simulink library "Susp_TwistBeam"  (R2025b)
settings: Solver=VariableStepAuto  StartTime=0.0  StopTime=10.0  RelTol=1e-3
undefined symbols (not defined in the file): Axle1D, AxleIn, Init, RaceFix, RaceSpin, TwistBeam, Visual, X, Y, Z
libraries: sm_lib x30, Suspension_Utilities x14, Linkage_Shock x2, fl_lib x2, nesl_utility x2, Linkage_Spring x2, Susp_TwistBeam_Components x2
(part 1 of 2)
Description:
  | Component of Simscape Vehicle Templates Library
  | 
  | Copyright 2018-2024 The MathWorks, Inc.
settings Model: Creator=mwalker  LastModifiedBy=smiller
settings SolverCC: AlgebraicLoopSolver=TrustRegion
settings DataIOCC: ReturnWorkspaceOutputs=off
settings DebuggingCC: UnconnectedInputMsg=warning  UnconnectedOutputMsg=warning  UnconnectedLineMsg=warning  ArithmeticOperatorsInVariantConditions=warning
settings ModelReferenceCC: EnableRefExpFcnMdlSchedulingChecks=on
settings SFSimCC: CustomCodeUndefinedFunction=UseInterfaceOnly
settings RTWCC: GPUComputeCapability=3.5

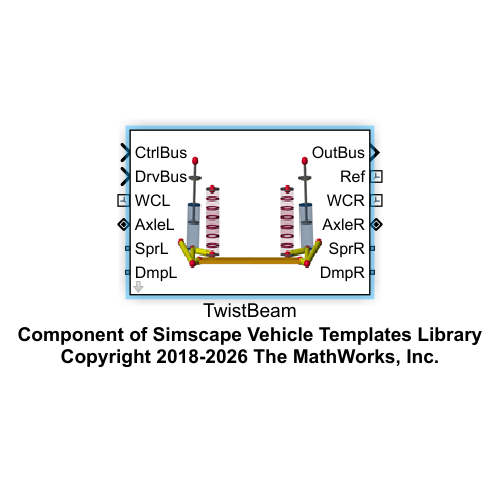
[thumbnail: Simulink's stored preview of the top-level diagram]
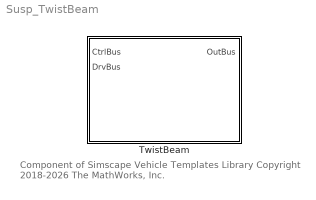
== system Susp_TwistBeam ==
  note: Component of Simscape Vehicle Templates Library
      | Copyright 2018-2026 The MathWorks, Inc.
  TwistBeam : Subsystem  VariantControl=LiveAxle  mask(Twist Beam Suspension){Init=Init.Axle2, hp_arm=TwistBeam.TrailingArm.sBody.Value, hp_dmp_top=TwistBeam.Damper.sTop.Value, hp_dmp_bot=TwistBeam.Damper.sBottom.Value, hp_spr_top=TwistBeam.Spring.sTop.Value, hp_spr_bot=TwistBeam.Spring.sBottom.Value, hp_beam=TwistBeam.Beam.sOutboard.Value, hp_whl_ctr=TwistBeam.TrailingArm.sWheelCentre.Value, Arm_to_Subframe=TwistBeam.Arm_to_Subframe, Damper_to_Subframe=TwistBeam.Damper_to_Subframe, Damper_to_Arm=TwistBeam.Damper_to_Arm, arm_mass=TwistBeam.TrailingArm.m.Value, axle_mass=TwistBeam.TrailingArm.mAxle.Value, axle_len=TwistBeam.TrailingArm.xAxle.Value, axle_whlc_to_bearing=TwistBeam.TrailingArm.xWCtoBearing.Value, beam_rho=TwistBeam.Beam.density.Value, beam_E=TwistBeam.Beam.E.Value, beam_nu=TwistBeam.Beam.nu.Value, beam_zeta=TwistBeam.Beam.zDamping.Value, xc_x=TwistBeam.Beam.xcX.Value, xc_z=TwistBeam.Beam.xcZ.Value, beam_numElements=TwistBeam.Beam.numElements.Value, opc_beam=Visual.part.opc, clr_beam=Visual.clr.orangedark, radius_axle=Visual.Axle.rad, clr_axle=Visual.Axle.clr, opc_axle=Visual.part.opc, clr_upr=Visual.UpperArm.clr, opc_upr=Visual.part.opc, piston_mass=TwistBeam.Shock.mPiston.Value, cyl_mass=TwistBeam.Shock.mCylinder.Value, damper_xmax=TwistBeam.Endstop.xMax.Value, damper_xmin=TwistBeam.Endstop.xMin.Value, spring_mass=TwistBeam.Spring.m.Value}
      mask prompts: Init "Initial Wheel Speed (rad/s)"; hp_arm "HP Arm to Body [xyz] (m)"; hp_dmp_top "HP Damper Top [xyz] (m)"; hp_dmp_bot "HP Damper Bottom [xyz] (m)"; hp_spr_top "HP Spring Top [xyz] (m)"; hp_spr_bot "HP Spring Bottom [xyz] (m)"; hp_beam "HP Beam Outboard [xyz] (m)"; hp_whl_ctr "HP Wheel Center [xyz] (m)"; Arm_to_Subframe "Arm to Subframe Connection (structure)"; Damper_to_Subframe "Damper to Subframe Connection"; Damper_to_Arm "Damper to Arm Connection"; arm_mass "Arm Mass (kg)"; axle_mass "Axle Mass (kg)"; axle_len "Axle Length (m)"; axle_whlc_to_bearing "Distance Wheel Ctr to Bearing (m)"; beam_rho "Beam Density (kg/m^3)"; beam_E "Young's Modulus (GPa)"; beam_nu "Poisson's Ratio"; beam_zeta "Damping Constant (sec)"; xc_x "Extrusion Points X (m)"; xc_z "Extrusion Points Z (m)"; beam_numElements "Number of Beam Elements"; opc_beam "Beam Opacity (0-1)"; clr_beam "Beam Color [RGB]"; radius_axle "Axle Radius (m)"; clr_axle "Axle Color [RGB]"; opc_axle "Axle Opacity (0-1)"; clr_upr "Bearing Color [RGB]"; opc_upr "Bearing Opacity (0-1)"; piston_mass "Piston Mass (kg)"; cyl_mass "Cylinder Mass (kg)"; damper_xmax "Upper Limit Bumpstop (m)"; damper_xmin "Lower Limit Bumpstop (m)"; spring_mass "Spring Mass (kg)"
      mask help: Models a twist beam suspension with independent connections for dampers and springs.
      mask TypeOptions axle_whlc_to_bearing:
      | Transform
      | sWheelCtrL/TranslationStandardOffset | Transform
      | sWheelCtrR/TranslationStandardOffset | Trailing
      | Arm L/axle_whlc_to_bearing | Trailing
      | Arm R/axle_whlc_to_bearing
      mask TypeOptions beam_rho: Beam/beam_rho
      mask TypeOptions beam_E: Beam/beam_E
      mask TypeOptions beam_nu: Beam/beam_nu
      mask TypeOptions beam_zeta: Beam/beam_zeta
      mask TypeOptions xc_x: Beam/xc_x
      mask TypeOptions xc_z: Beam/xc_z
      mask TypeOptions beam_numElements: Beam/beam_numElements
      mask TypeOptions opc_beam: Beam/opc_beam
      mask TypeOptions clr_beam: Beam/clr_beam
      mask DialogControl Container4 Prompt: Hardpoints
      mask DialogControl Container5 Prompt: Parts
      mask DialogControl Container7 Prompt: Visualization
      mask DialogControl Container6 Prompt: Shock
      mask Display: image('sm_car_vehicle_susp_twistbeam_IMAGE.png');

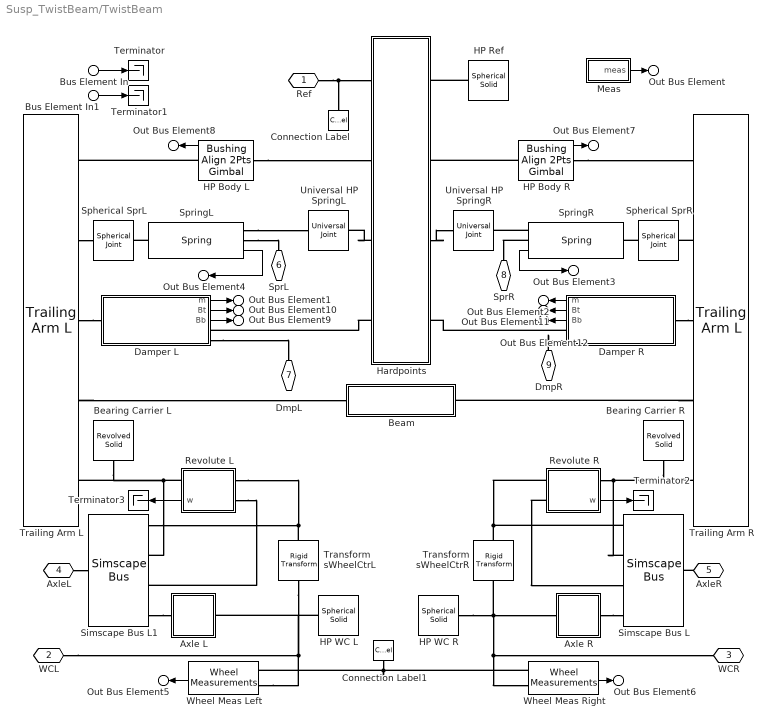
== system Susp_TwistBeam/TwistBeam ==
  Bus Element In1 : Inport  PortName=CtrlBus
  Bus Element In : Inport  Port=2  PortName=DrvBus
  Axle L : Subsystem
  Axle R : Subsystem
  Beam : Subsystem  mask(Leaf spring){popup_leftRight=Left, hp_beam=hp_beam, beam_rho=beam_rho, xc_x=xc_x, xc_z=xc_z, beam_E=beam_E, beam_nu=beam_nu, beam_zeta=beam_zeta, beam_numElements=beam_numElements, clr_beam=clr_beam, opc_beam=opc_beam}
      mask prompts: popup_leftRight "Left/Right"; hp_beam "HP Beam [xyz] (m)"; beam_rho "Beam Density (kg/m^3)"; xc_x "Extrusion Points X (m)"; xc_z "Extrusion Points Z (m)"; beam_E "Young's Modulus (GPa)"; beam_nu "Poisson's Ratio"; beam_zeta "Damping Constant (sec)"; beam_numElements "Number of Beam Elements"; clr_beam "Beam Color [RGB]"; opc_beam "Beam Opacity (0-1)"
      mask help: Models leaf spring using flexible body.
      mask init:
      | if(popup_leftRight == 1)
      |     rhs_susp = [1 1 1];
      | elseif(popup_leftRight == 2)
      |     rhs_susp = [1 -1 1];
      | end
      | 
      | beam_len = hp_beam(2)*2;
      mask TypeOptions popup_leftRight: Left | Right
      mask DialogControl cont_vis Prompt: Visualization
      mask Display: image('sm_car_vehicle_susp_leaf_spring_IMAGE.png')
  Bearing Carrier L : sm_lib/Body Elements/Revolved Solid  RevolutionCrossSection=[1.2 0.5;1.1 0.5;1.1 -0.5;1.2 -0.5].*[radius_axle 0.05]  RevolutionCrossSectionUnits=m  RevolutionExtent=Full  RevolutionAngle=180  RevolutionAngleUnits=deg  ExportConvexHullGeometry=off  InertiaType=CalculateFromGeometry  BasedOnType=Density  Density=1000  DensityUnits=kg/m^3  Mass=1  MassUnits=kg  CenterOfMass=[0 0 0]  CenterOfMassUnits=m  MomentsOfInertia=[1 1 1]  MomentsOfInertiaUnits=kg*m^2  ProductsOfInertia=[0 0 0]  ProductsOfInertiaUnits=kg*m^2  GraphicType=FromGeometry  MarkerShape=Sphere  MarkerSize=10  GraphicVisPropType=SimpleVisualProperties  GraphicDiffuseColor=clr_upr  GraphicOpacity=0.5  GraphicSpecularColor=[0.5 0.5 0.5 1.0]  GraphicAmbientColor=[0.15 0.15 0.15 1.0]  GraphicEmissiveColor=[0.0 0.0 0.0 1.0]  GraphicShininess=75  DoExposeReferenceFrame=on  SerializedFrames=<Frames/>
  Bearing Carrier R : sm_lib/Body Elements/Revolved Solid  RevolutionCrossSection=[1.2 0.5;1.1 0.5;1.1 -0.5;1.2 -0.5].*[radius_axle 0.05]  RevolutionCrossSectionUnits=m  RevolutionExtent=Full  RevolutionAngle=180  RevolutionAngleUnits=deg  ExportConvexHullGeometry=off  InertiaType=CalculateFromGeometry  BasedOnType=Density  Density=1000  DensityUnits=kg/m^3  Mass=1  MassUnits=kg  CenterOfMass=[0 0 0]  CenterOfMassUnits=m  MomentsOfInertia=[1 1 1]  MomentsOfInertiaUnits=kg*m^2  ProductsOfInertia=[0 0 0]  ProductsOfInertiaUnits=kg*m^2  GraphicType=FromGeometry  MarkerShape=Sphere  MarkerSize=10  GraphicVisPropType=SimpleVisualProperties  GraphicDiffuseColor=clr_upr  GraphicOpacity=0.5  GraphicSpecularColor=[0.5 0.5 0.5 1.0]  GraphicAmbientColor=[0.15 0.15 0.15 1.0]  GraphicEmissiveColor=[0.0 0.0 0.0 1.0]  GraphicShininess=75  DoExposeReferenceFrame=on  SerializedFrames=<Frames/>
  Connection Label : ConnectionLabel  Label=Ref
  Connection Label1 : ConnectionLabel  Label=Ref
  Damper L : Subsystem
      mask Display: image('sm_car_vehicle_linkage_shock_IMAGE.png');
  Damper R : Subsystem
      mask Display: image('sm_car_vehicle_linkage_shock_IMAGE.png');
  HP Body L : Suspension_Utilities/Bushing Align 2Pts Gimbal  VariantControl=Variant1  LabelModeActiveChoice=Bushing_Tr3Ro3  popup_leftRight=Left  hp_joint=hp_arm  Connection=Arm_to_Subframe  VariantLabel=Arm_to_Subframe.class.Value  checkbox_setTargets=off
      settings: AttributesFormatString=%<ActiveVariant>
  HP Body R : Suspension_Utilities/Bushing Align 2Pts Gimbal  VariantControl=Variant1  LabelModeActiveChoice=Bushing_Tr3Ro3  popup_leftRight=Right  hp_joint=hp_arm  Connection=Arm_to_Subframe  VariantLabel=Arm_to_Subframe.class.Value  checkbox_setTargets=off
      settings: AttributesFormatString=%<ActiveVariant>
  HP Ref : sm_lib/Body Elements/Spherical Solid  SphereRadius=Visual.hp.rad  SphereRadiusUnits=m  ExportEntireGeometry=off  InertiaType=CalculateFromGeometry  BasedOnType=Density  Density=1000  DensityUnits=kg/m^3  Mass=1  MassUnits=kg  CenterOfMass=[0 0 0]  CenterOfMassUnits=m  MomentsOfInertia=[1 1 1]  MomentsOfInertiaUnits=kg*m^2  ProductsOfInertia=[0 0 0]  ProductsOfInertiaUnits=kg*m^2  GraphicType=FromGeometry  MarkerShape=Sphere  MarkerSize=10  GraphicVisPropType=SimpleVisualProperties  GraphicDiffuseColor=Visual.hp.clr  GraphicOpacity=Visual.hp.opc  GraphicSpecularColor=[0.5 0.5 0.5 1.0]  GraphicAmbientColor=[0.15 0.15 0.15 1.0]  GraphicEmissiveColor=[0.0 0.0 0.0 1.0]  GraphicShininess=75  DoExposeReferenceFrame=on  SerializedFrames=<Frames/>
  HP WC L : sm_lib/Body Elements/Spherical Solid  SphereRadius=Visual.hp.rad  SphereRadiusUnits=m  ExportEntireGeometry=off  InertiaType=CalculateFromGeometry  BasedOnType=Density  Density=1000  DensityUnits=kg/m^3  Mass=1  MassUnits=kg  CenterOfMass=[0 0 0]  CenterOfMassUnits=m  MomentsOfInertia=[1 1 1]  MomentsOfInertiaUnits=kg*m^2  ProductsOfInertia=[0 0 0]  ProductsOfInertiaUnits=kg*m^2  GraphicType=FromGeometry  MarkerShape=Sphere  MarkerSize=10  GraphicVisPropType=SimpleVisualProperties  GraphicDiffuseColor=Visual.hp.clr  GraphicOpacity=Visual.hp.opc  GraphicSpecularColor=[0.5 0.5 0.5 1.0]  GraphicAmbientColor=[0.15 0.15 0.15 1.0]  GraphicEmissiveColor=[0.0 0.0 0.0 1.0]  GraphicShininess=75  DoExposeReferenceFrame=on  SerializedFrames=<Frames/>
  HP WC R : sm_lib/Body Elements/Spherical Solid  SphereRadius=Visual.hp.rad  SphereRadiusUnits=m  ExportEntireGeometry=off  InertiaType=CalculateFromGeometry  BasedOnType=Density  Density=1000  DensityUnits=kg/m^3  Mass=1  MassUnits=kg  CenterOfMass=[0 0 0]  CenterOfMassUnits=m  MomentsOfInertia=[1 1 1]  MomentsOfInertiaUnits=kg*m^2  ProductsOfInertia=[0 0 0]  ProductsOfInertiaUnits=kg*m^2  GraphicType=FromGeometry  MarkerShape=Sphere  MarkerSize=10  GraphicVisPropType=SimpleVisualProperties  GraphicDiffuseColor=Visual.hp.clr  GraphicOpacity=Visual.hp.opc  GraphicSpecularColor=[0.5 0.5 0.5 1.0]  GraphicAmbientColor=[0.15 0.15 0.15 1.0]  GraphicEmissiveColor=[0.0 0.0 0.0 1.0]  GraphicShininess=75  DoExposeReferenceFrame=on  SerializedFrames=<Frames/>
  Hardpoints : Subsystem
  Meas : Subsystem
  Revolute L : Subsystem  mask{whl_spd_init_jnt=Init.nWheel.Value(1)}
      mask prompts: whl_spd_init_jnt "Initial Wheel Speed (rad/s)"
      mask Display: image('sm_car_variant_revolute.png')
  Revolute R : Subsystem  mask{whl_spd_init_jnt=Init.nWheel.Value(2)}
      mask prompts: whl_spd_init_jnt "Initial Wheel Speed (rad/s)"
      mask Display: image('sm_car_variant_revolute.png')
  Simscape Bus L : SimscapeBus  HierarchyStrings=RaceSpin;RaceFix;Axle1D;AxleIn
  Simscape Bus L1 : SimscapeBus  HierarchyStrings=RaceSpin;RaceFix;Axle1D;AxleIn
  Spherical SprL : sm_lib/Joints/Spherical Joint  JointMode=Normal  CompositeWrenchDir=FollowerOnBase  CompositeWrenchFrame=BaseFrame  SenseConstraintForce=off  SenseConstraintTorque=off  SenseTotalForce=off  SenseTotalTorque=off  PositionTargetSpecify=off  PositionTargetPriority=High  PositionTargetRotationMethod=None  PositionTargetFollAlignAxisA=+X  PositionTargetBaseAlignAxisA=+Y  PositionTargetFollAlignAxisB=+Y  PositionTargetBaseAlignAxisB=+Z  PositionTargetRotationStandardAxis=+Z  PositionTargetRotationAngle=0.0  PositionTargetRotationAngleUnits=deg  PositionTargetRotationArbitraryAxis=[0 0 1]  PositionTargetRotationSequenceAxes=FollowerAxes  PositionTargetRotationSequence=XYX  PositionTargetRotationSequenceAngles=[0 0 0]  PositionTargetRotationSequenceAnglesUnits=deg  PositionTargetRotationMatrix=[1 0 0; 0 1 0; 0 0 1]  PositionTargetQuaternion=[1 0 0 0]  VelocityTargetSpecify=off  VelocityTargetPriority=High  VelocityTargetValue=[0 0 0]  VelocityTargetValueUnits=deg/s  VelocityTargetInFollowerFrame=on  EqPosRotationMethod=None  EqPosFollAlignAxisA=+X  EqPosBaseAlignAxisA=+Y  EqPosFollAlignAxisB=+Y  EqPosBaseAlignAxisB=+Z  EqPosRotationStandardAxis=+Z  EqPosRotationAngle=0.0  EqPosRotationAngleUnits=deg  EqPosRotationArbitraryAxis=[0 0 1]  EqPosRotationSequenceAxes=FollowerAxes  EqPosRotationSequence=XYX  EqPosRotationSequenceAngles=[0 0 0]  EqPosRotationSequenceAnglesUnits=deg  EqPosRotationMatrix=[1 0 0; 0 1 0; 0 0 1]  EqPosQuaternion=[1 0 0 0]  SpringStiffness=0  SpringStiffnessUnits=N*m/deg  DampingCoefficient=0  DampingCoefficientUnits=N*m/(deg/s)  LowerLimitSpecify=off  LowerLimitBound=15  LowerLimitBoundUnits=deg  LowerLimitStiffness=1e4  LowerLimitStiffnessUnits=N*m/deg  LowerLimitDamping=10  LowerLimitDampingUnits=N*m/(deg/s)  LowerLimitTransitionRegionWidth=0.1  LowerLimitTransitionRegionWidthUnits=deg  UpperLimitSpecify=off  UpperLimitBound=45  UpperLimitBoundUnits=deg  UpperLimitStiffness=1e4  UpperLimitStiffnessUnits=N*m/deg  UpperLimitDamping=10  UpperLimitDampingUnits=N*m/(deg/s)  UpperLimitTransitionRegionWidth=0.1  UpperLimitTransitionRegionWidthUnits=deg  TorqueActuationMode=NoTorque  ActuateTorqueX=off  ActuateTorqueY=off  ActuateTorqueZ=off  ActuateTorque=off  ActuationFrame=BaseFrame  SensePosition=off  SenseVelocityX=off  SenseVelocityY=off  SenseVelocityZ=off  SenseVelocity=off  SenseAccelerationX=off  SenseAccelerationY=off  SenseAccelerationZ=off  SenseAcceleration=off  SenseLowerLimitTorqueMag=off  SenseUpperLimitTorqueMag=off  SensingFrame=BaseFrame
  Spherical SprR : sm_lib/Joints/Spherical Joint  JointMode=Normal  CompositeWrenchDir=FollowerOnBase  CompositeWrenchFrame=BaseFrame  SenseConstraintForce=off  SenseConstraintTorque=off  SenseTotalForce=off  SenseTotalTorque=off  PositionTargetSpecify=off  PositionTargetPriority=High  PositionTargetRotationMethod=None  PositionTargetFollAlignAxisA=+X  PositionTargetBaseAlignAxisA=+Y  PositionTargetFollAlignAxisB=+Y  PositionTargetBaseAlignAxisB=+Z  PositionTargetRotationStandardAxis=+Z  PositionTargetRotationAngle=0.0  PositionTargetRotationAngleUnits=deg  PositionTargetRotationArbitraryAxis=[0 0 1]  PositionTargetRotationSequenceAxes=FollowerAxes  PositionTargetRotationSequence=XYX  PositionTargetRotationSequenceAngles=[0 0 0]  PositionTargetRotationSequenceAnglesUnits=deg  PositionTargetRotationMatrix=[1 0 0; 0 1 0; 0 0 1]  PositionTargetQuaternion=[1 0 0 0]  VelocityTargetSpecify=off  VelocityTargetPriority=High  VelocityTargetValue=[0 0 0]  VelocityTargetValueUnits=deg/s  VelocityTargetInFollowerFrame=on  EqPosRotationMethod=None  EqPosFollAlignAxisA=+X  EqPosBaseAlignAxisA=+Y  EqPosFollAlignAxisB=+Y  EqPosBaseAlignAxisB=+Z  EqPosRotationStandardAxis=+Z  EqPosRotationAngle=0.0  EqPosRotationAngleUnits=deg  EqPosRotationArbitraryAxis=[0 0 1]  EqPosRotationSequenceAxes=FollowerAxes  EqPosRotationSequence=XYX  EqPosRotationSequenceAngles=[0 0 0]  EqPosRotationSequenceAnglesUnits=deg  EqPosRotationMatrix=[1 0 0; 0 1 0; 0 0 1]  EqPosQuaternion=[1 0 0 0]  SpringStiffness=0  SpringStiffnessUnits=N*m/deg  DampingCoefficient=0  DampingCoefficientUnits=N*m/(deg/s)  LowerLimitSpecify=off  LowerLimitBound=15  LowerLimitBoundUnits=deg  LowerLimitStiffness=1e4  LowerLimitStiffnessUnits=N*m/deg  LowerLimitDamping=10  LowerLimitDampingUnits=N*m/(deg/s)  LowerLimitTransitionRegionWidth=0.1  LowerLimitTransitionRegionWidthUnits=deg  UpperLimitSpecify=off  UpperLimitBound=45  UpperLimitBoundUnits=deg  UpperLimitStiffness=1e4  UpperLimitStiffnessUnits=N*m/deg  UpperLimitDamping=10  UpperLimitDampingUnits=N*m/(deg/s)  UpperLimitTransitionRegionWidth=0.1  UpperLimitTransitionRegionWidthUnits=deg  TorqueActuationMode=NoTorque  ActuateTorqueX=off  ActuateTorqueY=off  ActuateTorqueZ=off  ActuateTorque=off  ActuationFrame=BaseFrame  SensePosition=off  SenseVelocityX=off  SenseVelocityY=off  SenseVelocityZ=off  SenseVelocity=off  SenseAccelerationX=off  SenseAccelerationY=off  SenseAccelerationZ=off  SenseAcceleration=off  SenseLowerLimitTorqueMag=off  SenseUpperLimitTorqueMag=off  SensingFrame=BaseFrame
  SpringL : Linkage_Spring/Spring  spring_mass=spring_mass  hp_spr_top=hp_spr_top  hp_spr_bot=hp_spr_bot  clr_conn_shock=Visual.hp.clr  opc_conn_shock=Visual.hp.opc  size_conn_shock=Visual.hp.rad  clr_spring_cyl=Visual.Spring.cyl.clr  opc_shock_cyl=Visual.Spring.cyl.opc  radius_shock_cyl=0.05  clr_spring_cap=Visual.Spring.cap.clr  opc_spring_cap=Visual.part.opc  clr_spring_coil=Visual.Spring.coil.clr  opc_spring_coil=Visual.Spring.coil.opc  cyl_cap_len_shock=Visual.Shock.cap.len
  SpringR : Linkage_Spring/Spring  spring_mass=spring_mass  hp_spr_top=hp_spr_top  hp_spr_bot=hp_spr_bot  clr_conn_shock=Visual.hp.clr  opc_conn_shock=Visual.hp.opc  size_conn_shock=Visual.hp.rad  clr_spring_cyl=Visual.Spring.cyl.clr  opc_shock_cyl=Visual.Spring.cyl.opc  radius_shock_cyl=0.05  clr_spring_cap=Visual.Spring.cap.clr  opc_spring_cap=Visual.part.opc  clr_spring_coil=Visual.Spring.coil.clr  opc_spring_coil=Visual.Spring.coil.opc  cyl_cap_len_shock=Visual.Shock.cap.len
  Terminator{,1..3} (4 alike) : Terminator
  Trailing Arm L : Susp_TwistBeam_Components/Trailing Arm L  VariantControl=Steer  popup_leftRight=Left  hp_body=hp_arm  hp_spr_bot=hp_spr_bot  hp_dam_bot=hp_dmp_bot  hp_wctr=hp_whl_ctr  hp_beam=hp_beam  axle_whlc_to_bearing=axle_whlc_to_bearing  rod_mass=arm_mass  clr_conn_rod=Visual.hp.clr  opc_conn_rod=Visual.hp.opc  size_conn_rod=Visual.hp.rad  clr_rod=Visual.UpperArm.clr  opc_rod=Visual.part.opc  radius_rod=Visual.UpperArm.rad
  Trailing Arm R : Susp_TwistBeam_Components/Trailing Arm L  VariantControl=Steer  popup_leftRight=Right  hp_body=hp_arm  hp_spr_bot=hp_spr_bot  hp_dam_bot=hp_dmp_bot  hp_wctr=hp_whl_ctr  hp_beam=hp_beam  axle_whlc_to_bearing=axle_whlc_to_bearing  rod_mass=arm_mass  clr_conn_rod=Visual.hp.clr  opc_conn_rod=Visual.hp.opc  size_conn_rod=Visual.hp.rad  clr_rod=Visual.UpperArm.clr  opc_rod=Visual.part.opc  radius_rod=Visual.UpperArm.rad
  Transform sWheelCtrL : sm_lib/Frames and Transforms/Rigid Transform  RotationMethod=None  FollAlignAxisA=+X  BaseAlignAxisA=+Y  FollAlignAxisB=+Y  BaseAlignAxisB=+Z  RotationStandardAxis=+X  RotationAngle=-90  RotationAngleUnits=deg  RotationArbitraryAxis=[0 0 1]  RotationSequenceAxes=FollowerAxes  RotationSequence=XYX  RotationSequenceAngles=[0 0 0]  RotationSequenceAnglesUnits=deg  RotationMatrix=[1 0 0; 0 1 0; 0 0 1]  Quaternion=[1 0 0 0]  TranslationMethod=StandardAxis  TranslationCartesianOffset=[0 0 0]  TranslationCartesianOffsetUnits=m  TranslationStandardAxis=-Z  TranslationStandardOffset=axle_whlc_to_bearing  TranslationStandardOffsetUnits=m  TranslationROffset=0  TranslationROffsetUnits=m  TranslationThetaOffset=0  TranslationThetaOffsetUnits=deg  TranslationZOffset=0  TranslationZOffsetUnits=m
  Transform sWheelCtrR : sm_lib/Frames and Transforms/Rigid Transform  RotationMethod=None  FollAlignAxisA=+X  BaseAlignAxisA=+Y  FollAlignAxisB=+Y  BaseAlignAxisB=+Z  RotationStandardAxis=+X  RotationAngle=-90  RotationAngleUnits=deg  RotationArbitraryAxis=[0 0 1]  RotationSequenceAxes=FollowerAxes  RotationSequence=XYX  RotationSequenceAngles=[0 0 0]  RotationSequenceAnglesUnits=deg  RotationMatrix=[1 0 0; 0 1 0; 0 0 1]  Quaternion=[1 0 0 0]  TranslationMethod=StandardAxis  TranslationCartesianOffset=[0 0 0]  TranslationCartesianOffsetUnits=m  TranslationStandardAxis=+Z  TranslationStandardOffset=axle_whlc_to_bearing  TranslationStandardOffsetUnits=m  TranslationROffset=0  TranslationROffsetUnits=m  TranslationThetaOffset=0  TranslationThetaOffsetUnits=deg  TranslationZOffset=0  TranslationZOffsetUnits=m
  Universal HP SpringL : sm_lib/Joints/Universal Joint  JointMode=Normal  CompositeWrenchDir=FollowerOnBase  CompositeWrenchFrame=BaseFrame  SenseConstraintForce=off  SenseConstraintTorque=off  SenseTotalForce=off  SenseTotalTorque=off  RxPositionTargetSpecify=off  RxPositionTargetPriority=High  RxPositionTargetValue=0  RxPositionTargetValueUnits=deg  RxVelocityTargetSpecify=off  RxVelocityTargetPriority=High  RxVelocityTargetValue=0  RxVelocityTargetValueUnits=deg/s  RxEquilibriumPosition=0  RxEquilibriumPositionUnits=deg  RxSpringStiffness=0  RxSpringStiffnessUnits=N*m/deg  RxDampingCoefficient=0  RxDampingCoefficientUnits=N*m/(deg/s)  RxLowerLimitSpecify=off  RxLowerLimitBound=-90  RxLowerLimitBoundUnits=deg  RxLowerLimitStiffness=1e4  RxLowerLimitStiffnessUnits=N*m/deg  RxLowerLimitDamping=10  RxLowerLimitDampingUnits=N*m/(deg/s)  RxLowerLimitTransitionRegionWidth=0.1  RxLowerLimitTransitionRegionWidthUnits=deg  RxUpperLimitSpecify=off  RxUpperLimitBound=90  RxUpperLimitBoundUnits=deg  RxUpperLimitStiffness=1e4  RxUpperLimitStiffnessUnits=N*m/deg  RxUpperLimitDamping=10  RxUpperLimitDampingUnits=N*m/(deg/s)  RxUpperLimitTransitionRegionWidth=0.1  RxUpperLimitTransitionRegionWidthUnits=deg  RxTorqueActuationMode=NoTorque  RxMotionActuationMode=ComputedMotion  RxSensePosition=off  RxSenseVelocity=off  RxSenseAcceleration=off  RxSenseTorqueForce=off  RxSenseLowerLimitTorqueForce=off  RxSenseUpperLimitTorqueForce=off  RyPositionTargetSpecify=off  RyPositionTargetPriority=High  RyPositionTargetValue=0  RyPositionTargetValueUnits=deg  RyVelocityTargetSpecify=off  RyVelocityTargetPriority=High  RyVelocityTargetValue=0  RyVelocityTargetValueUnits=deg/s  RyEquilibriumPosition=0  RyEquilibriumPositionUnits=deg  RySpringStiffness=0  RySpringStiffnessUnits=N*m/deg  RyDampingCoefficient=0  RyDampingCoefficientUnits=N*m/(deg/s)  RyLowerLimitSpecify=off  RyLowerLimitBound=-90  RyLowerLimitBoundUnits=deg  RyLowerLimitStiffness=1e4  RyLowerLimitStiffnessUnits=N*m/deg  RyLowerLimitDamping=10  RyLowerLimitDampingUnits=N*m/(deg/s)  RyLowerLimitTransitionRegionWidth=0.1  RyLowerLimitTransitionRegionWidthUnits=deg  RyUpperLimitSpecify=off  RyUpperLimitBound=90  RyUpperLimitBoundUnits=deg  RyUpperLimitStiffness=1e4  RyUpperLimitStiffnessUnits=N*m/deg  RyUpperLimitDamping=10  RyUpperLimitDampingUnits=N*m/(deg/s)  RyUpperLimitTransitionRegionWidth=0.1  RyUpperLimitTransitionRegionWidthUnits=deg  RyTorqueActuationMode=NoTorque  RyMotionActuationMode=ComputedMotion  RySensePosition=off  RySenseVelocity=off  RySenseAcceleration=off  RySenseTorqueForce=off  RySenseLowerLimitTorqueForce=off  RySenseUpperLimitTorqueForce=off
  Universal HP SpringR : sm_lib/Joints/Universal Joint  JointMode=Normal  CompositeWrenchDir=FollowerOnBase  CompositeWrenchFrame=BaseFrame  SenseConstraintForce=off  SenseConstraintTorque=off  SenseTotalForce=off  SenseTotalTorque=off  RxPositionTargetSpecify=off  RxPositionTargetPriority=High  RxPositionTargetValue=0  RxPositionTargetValueUnits=deg  RxVelocityTargetSpecify=off  RxVelocityTargetPriority=High  RxVelocityTargetValue=0  RxVelocityTargetValueUnits=deg/s  RxEquilibriumPosition=0  RxEquilibriumPositionUnits=deg  RxSpringStiffness=0  RxSpringStiffnessUnits=N*m/deg  RxDampingCoefficient=0  RxDampingCoefficientUnits=N*m/(deg/s)  RxLowerLimitSpecify=off  RxLowerLimitBound=-90  RxLowerLimitBoundUnits=deg  RxLowerLimitStiffness=1e4  RxLowerLimitStiffnessUnits=N*m/deg  RxLowerLimitDamping=10  RxLowerLimitDampingUnits=N*m/(deg/s)  RxLowerLimitTransitionRegionWidth=0.1  RxLowerLimitTransitionRegionWidthUnits=deg  RxUpperLimitSpecify=off  RxUpperLimitBound=90  RxUpperLimitBoundUnits=deg  RxUpperLimitStiffness=1e4  RxUpperLimitStiffnessUnits=N*m/deg  RxUpperLimitDamping=10  RxUpperLimitDampingUnits=N*m/(deg/s)  RxUpperLimitTransitionRegionWidth=0.1  RxUpperLimitTransitionRegionWidthUnits=deg  RxTorqueActuationMode=NoTorque  RxMotionActuationMode=ComputedMotion  RxSensePosition=off  RxSenseVelocity=off  RxSenseAcceleration=off  RxSenseTorqueForce=off  RxSenseLowerLimitTorqueForce=off  RxSenseUpperLimitTorqueForce=off  RyPositionTargetSpecify=off  RyPositionTargetPriority=High  RyPositionTargetValue=0  RyPositionTargetValueUnits=deg  RyVelocityTargetSpecify=off  RyVelocityTargetPriority=High  RyVelocityTargetValue=0  RyVelocityTargetValueUnits=deg/s  RyEquilibriumPosition=0  RyEquilibriumPositionUnits=deg  RySpringStiffness=0  RySpringStiffnessUnits=N*m/deg  RyDampingCoefficient=0  RyDampingCoefficientUnits=N*m/(deg/s)  RyLowerLimitSpecify=off  RyLowerLimitBound=-90  RyLowerLimitBoundUnits=deg  RyLowerLimitStiffness=1e4  RyLowerLimitStiffnessUnits=N*m/deg  RyLowerLimitDamping=10  RyLowerLimitDampingUnits=N*m/(deg/s)  RyLowerLimitTransitionRegionWidth=0.1  RyLowerLimitTransitionRegionWidthUnits=deg  RyUpperLimitSpecify=off  RyUpperLimitBound=90  RyUpperLimitBoundUnits=deg  RyUpperLimitStiffness=1e4  RyUpperLimitStiffnessUnits=N*m/deg  RyUpperLimitDamping=10  RyUpperLimitDampingUnits=N*m/(deg/s)  RyUpperLimitTransitionRegionWidth=0.1  RyUpperLimitTransitionRegionWidthUnits=deg  RyTorqueActuationMode=NoTorque  RyMotionActuationMode=ComputedMotion  RySensePosition=off  RySenseVelocity=off  RySenseAcceleration=off  RySenseTorqueForce=off  RySenseLowerLimitTorqueForce=off  RySenseUpperLimitTorqueForce=off
  Wheel Meas Left : Suspension_Utilities/Wheel Measurements  popup_leftRight=Left
  Wheel Meas Right : Suspension_Utilities/Wheel Measurements  popup_leftRight=Right
  Ref : PMIOPort  Side=Right
  WCL : PMIOPort  Port=2  Side=Left
  WCR : PMIOPort  Port=3  Side=Right
  AxleL : PMIOPort  Port=4  Side=Left
  AxleR : PMIOPort  Port=5  Side=Right
  SprL : PMIOPort  Port=6  Side=Left
  DmpL : PMIOPort  Port=7  Side=Left
  SprR : PMIOPort  Port=8  Side=Right
  DmpR : PMIOPort  Port=9  Side=Right
  Out Bus Element : Outport  VectorParamsAs1DForOutWhenUnconnected=off  PortName=OutBus  Element=Steer
  Out Bus Element1 : Outport  VectorParamsAs1DForOutWhenUnconnected=off  PortName=OutBus  Element=DamperL
  Out Bus Element2 : Outport  VectorParamsAs1DForOutWhenUnconnected=off  PortName=OutBus  Element=DamperR
  Out Bus Element3 : Outport  VectorParamsAs1DForOutWhenUnconnected=off  PortName=OutBus  Element=SpringR
  Out Bus Element4 : Outport  VectorParamsAs1DForOutWhenUnconnected=off  PortName=OutBus  Element=SpringL
  Out Bus Element5 : Outport  VectorParamsAs1DForOutWhenUnconnected=off  PortName=OutBus  Element=WhlL
  Out Bus Element6 : Outport  VectorParamsAs1DForOutWhenUnconnected=off  PortName=OutBus  Element=WhlR
  Out Bus Element7 : Outport  VectorParamsAs1DForOutWhenUnconnected=off  PortName=OutBus  Element=TAR
  Out Bus Element8 : Outport  VectorParamsAs1DForOutWhenUnconnected=off  PortName=OutBus  Element=TAL
  Out Bus Element9 : Outport  VectorParamsAs1DForOutWhenUnconnected=off  PortName=OutBus  Element=DprBL
  Out Bus Element10 : Outport  VectorParamsAs1DForOutWhenUnconnected=off  PortName=OutBus  Element=DprTL
  Out Bus Element11 : Outport  VectorParamsAs1DForOutWhenUnconnected=off  PortName=OutBus  Element=DprTR
  Out Bus Element12 : Outport  VectorParamsAs1DForOutWhenUnconnected=off  PortName=OutBus  Element=DprBR
  wires:
  Bus Element In1/1 -> Terminator1/1
  Meas/1(meas) -> Out Bus Element/1
  Bus Element In/1 -> Terminator/1
  Revolute R/1(w) -> Terminator2/1
  Revolute L/1(w) -> Terminator3/1
  SpringR/1 -> Out Bus Element3/1
  SpringL/1 -> Out Bus Element4/1
  Damper L/1(m) -> Out Bus Element1/1
  Damper R/1(m) -> Out Bus Element2/1
  Wheel Meas Left/1 -> Out Bus Element5/1
  Wheel Meas Right/1 -> Out Bus Element6/1
  HP Body R/1 -> Out Bus Element7/1
  HP Body L/1 -> Out Bus Element8/1
  Damper L/3(Bb) -> Out Bus Element9/1
  Damper L/2(Bt) -> Out Bus Element10/1
  Damper R/2(Bt) -> Out Bus Element11/1
  Damper R/3(Bb) -> Out Bus Element12/1
  connections:
  Trailing Arm R/LConn4 -- Beam/RConn1
  Simscape Bus L/LConn2 -- Trailing Arm R/LConn5 -- Bearing Carrier R/RConn1 -- Revolute R/RConn1
  Revolute L/RConn1 -- Bearing Carrier L/RConn1 -- Trailing Arm L/LConn5 -- Simscape Bus L1/LConn2
  AxleR/RConn1 -- Simscape Bus L/RConn1
  Revolute R/LConn2 -- Simscape Bus L/LConn1 -- Transform sWheelCtrR/RConn1
  Revolute R/LConn1 -- Simscape Bus L/LConn3
  AxleL/RConn1 -- Simscape Bus L1/RConn1
  Revolute L/LConn2 -- Simscape Bus L1/LConn1 -- Transform sWheelCtrL/RConn1
  Revolute L/LConn1 -- Simscape Bus L1/LConn3
  Simscape Bus L1/LConn4 -- Axle L/RConn1
  Trailing Arm L/LConn2 -- Spherical SprL/LConn1
  Trailing Arm L/LConn4 -- Beam/LConn1
  SpringL/RConn1 -- SprL/RConn1
  SpringL/LConn1 -- Spherical SprL/RConn1
  SpringL/RConn2 -- Universal HP SpringL/RConn1
  SpringR/RConn2 -- Universal HP SpringR/RConn1
  Spherical SprR/RConn1 -- SpringR/LConn1
  Trailing Arm R/LConn2 -- Spherical SprR/LConn1
  SpringR/RConn1 -- SprR/RConn1
  HP Body R/RConn1 -- Trailing Arm R/LConn1
  HP Body L/RConn1 -- Trailing Arm L/LConn1
  Ref/RConn1 -- Hardpoints/LConn1 -- Connection Label/LConn1
  HP Body L/LConn1 -- Hardpoints/LConn2
  HP Body R/LConn1 -- Hardpoints/RConn2
  Hardpoints/LConn3 -- Universal HP SpringL/LConn1
  Hardpoints/RConn3 -- Universal HP SpringR/LConn1
  HP Ref/RConn1 -- Hardpoints/RConn1
  Hardpoints/LConn4 -- Damper L/RConn1
  Trailing Arm L/LConn3 -- Damper L/LConn1
  Damper L/RConn2 -- DmpL/RConn1
  Damper R/RConn1 -- Hardpoints/RConn4
  Damper R/LConn1 -- Trailing Arm R/LConn3
  DmpR/RConn1 -- Damper R/RConn2
  Connection Label1/LConn1 -- Wheel Meas Right/LConn1 -- Wheel Meas Left/LConn1
  Wheel Meas Left/LConn2 -- HP WC L/RConn1 -- Transform sWheelCtrL/LConn1 -- Axle L/LConn1 -- WCL/RConn1
  HP WC R/RConn1 -- WCR/RConn1 -- Wheel Meas Right/LConn2 -- Axle R/LConn1 -- Transform sWheelCtrR/LConn1
  Axle R/RConn1 -- Simscape Bus L/LConn4

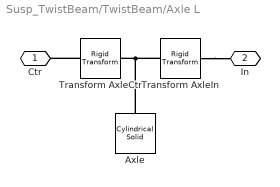
== system Susp_TwistBeam/TwistBeam/Axle L ==
  Axle : sm_lib/Body Elements/Cylindrical Solid  CylinderRadius=radius_axle  CylinderRadiusUnits=m  CylinderLength=axle_len  CylinderLengthUnits=m  ExportEntireGeometry=off  InertiaType=CalculateFromGeometry  BasedOnType=Mass  Density=7000  DensityUnits=kg/m^3  Mass=axle_mass  MassUnits=kg  CenterOfMass=[0 0 0]  CenterOfMassUnits=m  MomentsOfInertia=[1 1 1]  MomentsOfInertiaUnits=kg*m^2  ProductsOfInertia=[0 0 0]  ProductsOfInertiaUnits=kg*m^2  GraphicType=FromGeometry  MarkerShape=Sphere  MarkerSize=10  GraphicVisPropType=SimpleVisualProperties  GraphicDiffuseColor=clr_axle  GraphicOpacity=opc_axle  GraphicSpecularColor=[0.5 0.5 0.5 1.0]  GraphicAmbientColor=[0.15 0.15 0.15 1.0]  GraphicEmissiveColor=[0.0 0.0 0.0 1.0]  GraphicShininess=75  DoExposeReferenceFrame=on  SerializedFrames=<Frames/>
  Transform AxleCtr : sm_lib/Frames and Transforms/Rigid Transform  RotationMethod=None  FollAlignAxisA=+X  BaseAlignAxisA=+Y  FollAlignAxisB=+Y  BaseAlignAxisB=+Z  RotationStandardAxis=+Z  RotationAngle=0  RotationAngleUnits=deg  RotationArbitraryAxis=[0 0 1]  RotationSequenceAxes=FollowerAxes  RotationSequence=XYX  RotationSequenceAngles=[0 0 0]  RotationSequenceAnglesUnits=deg  RotationMatrix=[1 0 0; 0 1 0; 0 0 1]  Quaternion=[1 0 0 0]  TranslationMethod=StandardAxis  TranslationCartesianOffset=[0 0 0]  TranslationCartesianOffsetUnits=m  TranslationStandardAxis=-Z  TranslationStandardOffset=axle_len/2  TranslationStandardOffsetUnits=m  TranslationROffset=0  TranslationROffsetUnits=m  TranslationThetaOffset=0  TranslationThetaOffsetUnits=deg  TranslationZOffset=0  TranslationZOffsetUnits=m
  Transform AxleIn : sm_lib/Frames and Transforms/Rigid Transform  RotationMethod=None  FollAlignAxisA=+X  BaseAlignAxisA=+Y  FollAlignAxisB=+Y  BaseAlignAxisB=+Z  RotationStandardAxis=+Z  RotationAngle=0  RotationAngleUnits=deg  RotationArbitraryAxis=[0 0 1]  RotationSequenceAxes=FollowerAxes  RotationSequence=XYX  RotationSequenceAngles=[0 0 0]  RotationSequenceAnglesUnits=deg  RotationMatrix=[1 0 0; 0 1 0; 0 0 1]  Quaternion=[1 0 0 0]  TranslationMethod=StandardAxis  TranslationCartesianOffset=[0 0 0]  TranslationCartesianOffsetUnits=m  TranslationStandardAxis=-Z  TranslationStandardOffset=axle_len/2  TranslationStandardOffsetUnits=m  TranslationROffset=0  TranslationROffsetUnits=m  TranslationThetaOffset=0  TranslationThetaOffsetUnits=deg  TranslationZOffset=0  TranslationZOffsetUnits=m
  Ctr : PMIOPort  Side=Left
  In : PMIOPort  Port=2  Side=Right
  connections:
  Axle/RConn1 -- Transform AxleCtr/RConn1 -- Transform AxleIn/LConn1
  Transform AxleCtr/LConn1 -- Ctr/RConn1
  Transform AxleIn/RConn1 -- In/RConn1

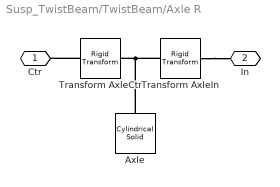
== system Susp_TwistBeam/TwistBeam/Axle R ==
  Axle : sm_lib/Body Elements/Cylindrical Solid  CylinderRadius=radius_axle  CylinderRadiusUnits=m  CylinderLength=axle_len  CylinderLengthUnits=m  ExportEntireGeometry=off  InertiaType=CalculateFromGeometry  BasedOnType=Mass  Density=7000  DensityUnits=kg/m^3  Mass=axle_mass  MassUnits=kg  CenterOfMass=[0 0 0]  CenterOfMassUnits=m  MomentsOfInertia=[1 1 1]  MomentsOfInertiaUnits=kg*m^2  ProductsOfInertia=[0 0 0]  ProductsOfInertiaUnits=kg*m^2  GraphicType=FromGeometry  MarkerShape=Sphere  MarkerSize=10  GraphicVisPropType=SimpleVisualProperties  GraphicDiffuseColor=clr_axle  GraphicOpacity=opc_axle  GraphicSpecularColor=[0.5 0.5 0.5 1.0]  GraphicAmbientColor=[0.15 0.15 0.15 1.0]  GraphicEmissiveColor=[0.0 0.0 0.0 1.0]  GraphicShininess=75  DoExposeReferenceFrame=on  SerializedFrames=<Frames/>
  Transform AxleCtr : sm_lib/Frames and Transforms/Rigid Transform  RotationMethod=None  FollAlignAxisA=+X  BaseAlignAxisA=+Y  FollAlignAxisB=+Y  BaseAlignAxisB=+Z  RotationStandardAxis=+Z  RotationAngle=0  RotationAngleUnits=deg  RotationArbitraryAxis=[0 0 1]  RotationSequenceAxes=FollowerAxes  RotationSequence=XYX  RotationSequenceAngles=[0 0 0]  RotationSequenceAnglesUnits=deg  RotationMatrix=[1 0 0; 0 1 0; 0 0 1]  Quaternion=[1 0 0 0]  TranslationMethod=StandardAxis  TranslationCartesianOffset=[0 0 0]  TranslationCartesianOffsetUnits=m  TranslationStandardAxis=-Z  TranslationStandardOffset=-axle_len/2  TranslationStandardOffsetUnits=m  TranslationROffset=0  TranslationROffsetUnits=m  TranslationThetaOffset=0  TranslationThetaOffsetUnits=deg  TranslationZOffset=0  TranslationZOffsetUnits=m
  Transform AxleIn : sm_lib/Frames and Transforms/Rigid Transform  RotationMethod=None  FollAlignAxisA=+X  BaseAlignAxisA=+Y  FollAlignAxisB=+Y  BaseAlignAxisB=+Z  RotationStandardAxis=+Z  RotationAngle=0  RotationAngleUnits=deg  RotationArbitraryAxis=[0 0 1]  RotationSequenceAxes=FollowerAxes  RotationSequence=XYX  RotationSequenceAngles=[0 0 0]  RotationSequenceAnglesUnits=deg  RotationMatrix=[1 0 0; 0 1 0; 0 0 1]  Quaternion=[1 0 0 0]  TranslationMethod=StandardAxis  TranslationCartesianOffset=[0 0 0]  TranslationCartesianOffsetUnits=m  TranslationStandardAxis=-Z  TranslationStandardOffset=-axle_len/2  TranslationStandardOffsetUnits=m  TranslationROffset=0  TranslationROffsetUnits=m  TranslationThetaOffset=0  TranslationThetaOffsetUnits=deg  TranslationZOffset=0  TranslationZOffsetUnits=m
  Ctr : PMIOPort  Side=Left
  In : PMIOPort  Port=2  Side=Right
  connections:
  Transform AxleIn/RConn1 -- In/RConn1
  Transform AxleCtr/LConn1 -- Ctr/RConn1
  Transform AxleCtr/RConn1 -- Axle/RConn1 -- Transform AxleIn/LConn1

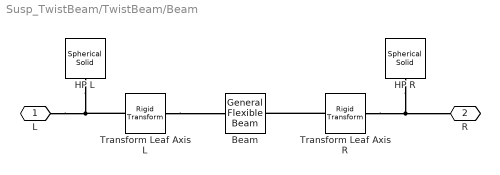
== system Susp_TwistBeam/TwistBeam/Beam ==
  Beam : sm_lib/Body Elements/Flexible Bodies/Beams/General Flexible Beam  ExtrusionCrossSection=[xc_x' xc_z']  ExtrusionCrossSectionUnits=m  ExtrusionLength=beam_len  ExtrusionLengthUnits=m  StiffnessAndInertiaType=CalculateFromGeometry  Density=beam_rho  DensityUnits=kg/m^3  ModuliType=YoungsPoissons  YoungsModulus=beam_E  YoungsModulusUnits=GPa  PoissonsRatio=beam_nu  ShearModulus=26  ShearModulusUnits=GPa  GeometricCentroid=[0 0]  GeometricCentroidUnits=m  BendingCentroid=[0 0]  BendingCentroidUnits=m  ShearCenter=[0 0]  ShearCenterUnits=m  AxialRigidity=1  AxialRigidityUnits=Pa*m^2  FlexuralRigidity=[1 1]  FlexuralRigidityUnits=Pa*m^4  CrossFlexuralRigidity=0  CrossFlexuralRigidityUnits=Pa*m^4  TorsionalRigidity=1  TorsionalRigidityUnits=Pa*m^4  CenterOfMass=[0 0]  CenterOfMassUnits=m  MassPerUnitLength=1  MassPerUnitLengthUnits=kg/m  MassMomentOfInertiaDensity=[1 1]  MassMomentOfInertiaDensityUnits=kg*m  MassProductOfInertiaDensity=0  MassProductOfInertiaDensityUnits=kg*m  DampingType=Proportional  ProportionalDampingAlpha=0  ProportionalDampingAlphaUnits=1/s  ProportionalDampingBeta=beam_zeta  ProportionalDampingBetaUnits=s  UniformModalDampingRatio=0.01  NumElements=beam_numElements  ReferenceConditionsType=LinearizedMeanAxes  DoExposeReferenceFrame=off  ReductionType=None  NumRetainedModes=1  GraphicType=FromGeometry  GraphicVisPropType=SimpleVisualProperties  GraphicDiffuseColor=clr_beam  GraphicOpacity=opc_beam  GraphicSpecularColor=[0.5 0.5 0.5 1.0]  GraphicAmbientColor=[0.15 0.15 0.15 1.0]  GraphicEmissiveColor=[0.0 0.0 0.0 1.0]  GraphicShininess=75  DoExposeZminFrame=on  DoExposeZmaxFrame=on  SerializedFrames=<Frames/>
  HP L : sm_lib/Body Elements/Spherical Solid  SphereRadius=Visual.hp.rad  SphereRadiusUnits=m  ExportEntireGeometry=off  InertiaType=CalculateFromGeometry  BasedOnType=Density  Density=1000  DensityUnits=kg/m^3  Mass=1  MassUnits=kg  CenterOfMass=[0 0 0]  CenterOfMassUnits=m  MomentsOfInertia=[1 1 1]  MomentsOfInertiaUnits=kg*m^2  ProductsOfInertia=[0 0 0]  ProductsOfInertiaUnits=kg*m^2  GraphicType=FromGeometry  MarkerShape=Sphere  MarkerSize=10  GraphicVisPropType=SimpleVisualProperties  GraphicDiffuseColor=Visual.hp.clr  GraphicOpacity=Visual.hp.opc  GraphicSpecularColor=[0.5 0.5 0.5 1.0]  GraphicAmbientColor=[0.15 0.15 0.15 1.0]  GraphicEmissiveColor=[0.0 0.0 0.0 1.0]  GraphicShininess=75  DoExposeReferenceFrame=on  SerializedFrames=<Frames/>
  HP R : sm_lib/Body Elements/Spherical Solid  SphereRadius=Visual.hp.rad  SphereRadiusUnits=m  ExportEntireGeometry=off  InertiaType=CalculateFromGeometry  BasedOnType=Density  Density=1000  DensityUnits=kg/m^3  Mass=1  MassUnits=kg  CenterOfMass=[0 0 0]  CenterOfMassUnits=m  MomentsOfInertia=[1 1 1]  MomentsOfInertiaUnits=kg*m^2  ProductsOfInertia=[0 0 0]  ProductsOfInertiaUnits=kg*m^2  GraphicType=FromGeometry  MarkerShape=Sphere  MarkerSize=10  GraphicVisPropType=SimpleVisualProperties  GraphicDiffuseColor=Visual.hp.clr  GraphicOpacity=Visual.hp.opc  GraphicSpecularColor=[0.5 0.5 0.5 1.0]  GraphicAmbientColor=[0.15 0.15 0.15 1.0]  GraphicEmissiveColor=[0.0 0.0 0.0 1.0]  GraphicShininess=75  DoExposeReferenceFrame=on  SerializedFrames=<Frames/>
  Transform Leaf Axis L : sm_lib/Frames and Transforms/Rigid Transform  RotationMethod=RotationSequence  FollAlignAxisA=-Z  BaseAlignAxisA=+X  FollAlignAxisB=+Y  BaseAlignAxisB=+Y  RotationStandardAxis=+X  RotationAngle=90  RotationAngleUnits=deg  RotationArbitraryAxis=[0 0 1]  RotationSequenceAxes=FollowerAxes  RotationSequence=XZX  RotationSequenceAngles=[90 0 0]  RotationSequenceAnglesUnits=deg  RotationMatrix=[1 0 0; 0 1 0; 0 0 1]  Quaternion=[1 0 0 0]  TranslationMethod=None  TranslationCartesianOffset=[0 0 0]  TranslationCartesianOffsetUnits=m  TranslationStandardAxis=+Z  TranslationStandardOffset=0  TranslationStandardOffsetUnits=m  TranslationROffset=0  TranslationROffsetUnits=m  TranslationThetaOffset=0  TranslationThetaOffsetUnits=deg  TranslationZOffset=0  TranslationZOffsetUnits=m
  Transform Leaf Axis R : sm_lib/Frames and Transforms/Rigid Transform  RotationMethod=RotationSequence  FollAlignAxisA=-Z  BaseAlignAxisA=+X  FollAlignAxisB=+Y  BaseAlignAxisB=+Y  RotationStandardAxis=+X  RotationAngle=90  RotationAngleUnits=deg  RotationArbitraryAxis=[0 0 1]  RotationSequenceAxes=FollowerAxes  RotationSequence=XZX  RotationSequenceAngles=[90 0 0]  RotationSequenceAnglesUnits=deg  RotationMatrix=[1 0 0; 0 1 0; 0 0 1]  Quaternion=[1 0 0 0]  TranslationMethod=None  TranslationCartesianOffset=[0 0 0]  TranslationCartesianOffsetUnits=m  TranslationStandardAxis=+Z  TranslationStandardOffset=0  TranslationStandardOffsetUnits=m  TranslationROffset=0  TranslationROffsetUnits=m  TranslationThetaOffset=0  TranslationThetaOffsetUnits=deg  TranslationZOffset=0  TranslationZOffsetUnits=m
  L : PMIOPort  Side=Left
  R : PMIOPort  Port=2  Side=Right
  connections:
  Transform Leaf Axis R/RConn1 -- Beam/RConn1
  Transform Leaf Axis L/RConn1 -- Beam/LConn1
  Transform Leaf Axis R/LConn1 -- R/RConn1 -- HP R/RConn1
  Transform Leaf Axis L/LConn1 -- L/RConn1 -- HP L/RConn1

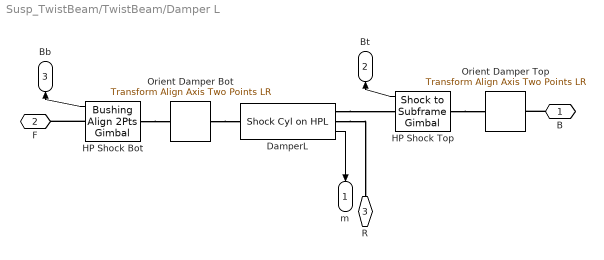
== system Susp_TwistBeam/TwistBeam/Damper L ==
  DamperL : Linkage_Shock/Shock Cyl on HPL  shock_pist_mass=piston_mass  shock_cyl_mass=cyl_mass  hp_spr_top=hp_dmp_top  hp_spr_bot=hp_dmp_bot  up_lim_bumpstop=damper_xmax  low_lim_bumpstop=damper_xmin  clr_conn_shock=Visual.hp.clr  opc_conn_shock=Visual.hp.opc  size_conn_shock=Visual.hp.rad  clr_shock_cyl=Visual.clr.blue  opc_shock_cyl=Visual.part.opc  radius_shock_cyl=0.05  clr_shock_piston=Visual.clr.gray  opc_shock_piston=Visual.part.opc  clr_shock_bumpstop=Visual.clr.yellowpale  opc_shock_bumpstop=Visual.part.opc  deadvol_len_shock_cyl=Visual.Shock.dead_length  piston_len_shock=Visual.Shock.piston.len  cyl_cap_len_shock=Visual.Shock.cap.len  bumpstop_len_shock=Visual.Shock.bumpstop.len
  HP Shock Bot : Suspension_Utilities/Bushing Align 2Pts Gimbal  VariantControl=Variant1  LabelModeActiveChoice=Bushing_Tr3Ro3  popup_leftRight=Left  hp_joint=hp_dmp_bot  Connection=Damper_to_Arm  VariantLabel=Damper_to_Arm.class.Value  checkbox_setTargets=off
      settings: AttributesFormatString=%<ActiveVariant>
  HP Shock Top : Suspension_Utilities/Shock to Subframe Gimbal  VariantControl=Variant1  LabelModeActiveChoice=Bushing_Tr3Ro3  popup_leftRight=Left  Connection=Damper_to_Subframe  VariantLabel=Damper_to_Subframe.class.Value  checkbox_setTargets=on
      settings: AttributesFormatString=%<ActiveVariant>
  Orient Damper Bot : Suspension_Utilities/Transform Align Axis Two Points LR  popup_leftRight=Left  hp_spr_top=hp_dmp_top  hp_spr_bot=hp_dmp_bot
  Orient Damper Top : Suspension_Utilities/Transform Align Axis Two Points LR  popup_leftRight=Left  hp_spr_top=hp_dmp_top  hp_spr_bot=hp_dmp_bot
  B : PMIOPort  Side=Right
  F : PMIOPort  Port=2  Side=Left
  R : PMIOPort  Port=3  Side=Right
  m : Outport
  Bt : Outport  Port=2
  Bb : Outport  Port=3
  wires:
  DamperL/1 -> m/1
  HP Shock Bot/1 -> Bb/1
  HP Shock Top/1 -> Bt/1
  connections:
  B/RConn1 -- Orient Damper Top/LConn1
  HP Shock Top/LConn1 -- Orient Damper Top/RConn1
  Orient Damper Bot/RConn1 -- DamperL/LConn1
  DamperL/RConn2 -- HP Shock Top/RConn1
  HP Shock Bot/RConn1 -- F/RConn1
  HP Shock Bot/LConn1 -- Orient Damper Bot/LConn1
  DamperL/RConn1 -- R/RConn1

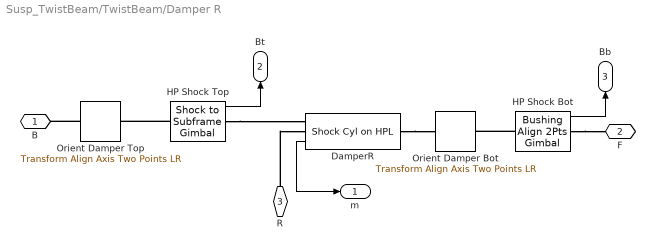
== system Susp_TwistBeam/TwistBeam/Damper R ==
  DamperR : Linkage_Shock/Shock Cyl on HPL  shock_pist_mass=piston_mass  shock_cyl_mass=cyl_mass  hp_spr_top=hp_dmp_top  hp_spr_bot=hp_dmp_bot  up_lim_bumpstop=damper_xmax  low_lim_bumpstop=damper_xmin  clr_conn_shock=Visual.hp.clr  opc_conn_shock=Visual.hp.opc  size_conn_shock=Visual.hp.rad  clr_shock_cyl=Visual.clr.blue  opc_shock_cyl=Visual.part.opc  radius_shock_cyl=0.05  clr_shock_piston=Visual.clr.gray  opc_shock_piston=Visual.part.opc  clr_shock_bumpstop=Visual.clr.yellowpale  opc_shock_bumpstop=Visual.part.opc  deadvol_len_shock_cyl=Visual.Shock.dead_length  piston_len_shock=Visual.Shock.piston.len  cyl_cap_len_shock=Visual.Shock.cap.len  bumpstop_len_shock=Visual.Shock.bumpstop.len
  HP Shock Bot : Suspension_Utilities/Bushing Align 2Pts Gimbal  VariantControl=Variant1  LabelModeActiveChoice=Bushing_Tr3Ro3  popup_leftRight=Right  hp_joint=hp_dmp_bot  Connection=Damper_to_Arm  VariantLabel=Damper_to_Arm.class.Value  checkbox_setTargets=on
      settings: AttributesFormatString=%<ActiveVariant>
  HP Shock Top : Suspension_Utilities/Shock to Subframe Gimbal  VariantControl=Variant1  LabelModeActiveChoice=Bushing_Tr3Ro3  popup_leftRight=Right  Connection=Damper_to_Subframe  VariantLabel=Damper_to_Subframe.class.Value  checkbox_setTargets=off
      settings: AttributesFormatString=%<ActiveVariant>
  Orient Damper Bot : Suspension_Utilities/Transform Align Axis Two Points LR  popup_leftRight=Left  hp_spr_top=hp_dmp_top  hp_spr_bot=hp_dmp_bot
  Orient Damper Top : Suspension_Utilities/Transform Align Axis Two Points LR  popup_leftRight=Right  hp_spr_top=hp_dmp_top  hp_spr_bot=hp_dmp_bot
  B : PMIOPort  Side=Right
  F : PMIOPort  Port=2  Side=Left
  R : PMIOPort  Port=3  Side=Right
  m : Outport
  Bt : Outport  Port=2
  Bb : Outport  Port=3
  wires:
  DamperR/1 -> m/1
  HP Shock Bot/1 -> Bb/1
  HP Shock Top/1 -> Bt/1
  connections:
  DamperR/LConn1 -- Orient Damper Bot/RConn1
  HP Shock Top/RConn1 -- DamperR/RConn2
  HP Shock Top/LConn1 -- Orient Damper Top/RConn1
  Orient Damper Top/LConn1 -- B/RConn1
  HP Shock Bot/RConn1 -- F/RConn1
  HP Shock Bot/LConn1 -- Orient Damper Bot/LConn1
  R/RConn1 -- DamperR/RConn1
